simulink model "prjKGr_2021"  (R2023a)
settings: Solver=FixedStepAuto  StartTime=0.0  StopTime=60*5  FixedStep=0.002  RelTol=1e-3  EnableMultiTasking=on
values from neighbouring files (symbols this model uses):
  a0 = pi * (d0 / 2)^2    (= 1.55528471307e-05)    [calculate_matrix.m]    (also in equilibrum_h.m; param_G3.m)
  A0 = pi * (Di / 2)^2    (= 0.00155179165474)    [calculate_matrix.m]    (also in equilibrum_h.m; param_G3.m)
  A1 = pi * (Di / 2)^2    (= 0.00155179165474)    [calculate_matrix.m]    (also in equilibrum_h.m; param_G3.m)
  a1 = pi * (d1 / 2)^2    (= 2.42471809941e-05)    [calculate_matrix.m]    (also in equilibrum_h.m; param_G3.m)
  a2 = pi * (d0 / 2)^2    (= 1.55528471307e-05)    [calculate_matrix.m]    (also in equilibrum_h.m; param_G3.m)
  A2 = pi * (Di / 2)^2    (= 0.00155179165474)    [calculate_matrix.m]    (also in equilibrum_h.m; param_G3.m)
  A3 = pi * (Di / 2)^2    (= 0.00155179165474)    [calculate_matrix.m]    (also in equilibrum_h.m; param_G3.m)
  a3 = pi * (d1 / 2)^2    (= 2.42471809941e-05)    [calculate_matrix.m]    (also in equilibrum_h.m; param_G3.m)
  g = 9.8    [calculate_matrix.m]    (also in equilibrum_h.m; param_G3.m = 9.81)
  gamma = 0.61    [calculate_matrix.m]    (also in equilibrum_h.m; param_G3.m)
  h0eq = 0.1220    (= 0.122)    [param_G3.m]
  h1eq = 0.1286    [param_G3.m]
  h2eq = 0.1077    [param_G3.m]
  h3eq = 0.1252    [param_G3.m]
  K = -Quuinv*Qux    [param_G3.m]
  k0 = 3.9e-6    (= 3.9e-06)    [calculate_matrix.m]    (also in equilibrum_h.m; param_G3.m)
  k1 = 4.15e-6    (= 4.15e-06)    [calculate_matrix.m]    (also in equilibrum_h.m; param_G3.m)
  v0eq = 9.5    [param_G3.m]
  v1eq = 9.5    [param_G3.m]
undefined symbols (not defined in the file or in its folder): HIL
libraries: quarc_library x3
settings Model: Creator=Simulatore DELAB  LastModifiedBy=CRS
settings SolverCC: PositivePriorityOrder=on  AutoInsertRateTranBlk=on
settings DebuggingCC: UnconnectedInputMsg=warning  UnconnectedOutputMsg=warning  UnconnectedLineMsg=warning
settings ModelReferenceCC: EnableRefExpFcnMdlSchedulingChecks=on
settings RTWCC: Description=QUARC Win64 Target Using Toolchain  SystemTargetFile=quarc_win64.tlc  Toolchain=QUARC win64 | nmake (64-bit Windows)  BuildConfiguration=Faster Runs  DLArmComputeVersion=19.05
settings STFCustomTargetCC: SystemTargetFile=quarc_win64.tlc
settings GRTTargetCC: ParMdlRefBuildCompliant=off  CompOptLevelCompliant=off  CombineOutputUpdateFcns=off  MatFileLogging=off  CPPClassGenCompliant=off  GRTInterface=on  ExtMode=on  ExtModeMexFile=quarc_comm

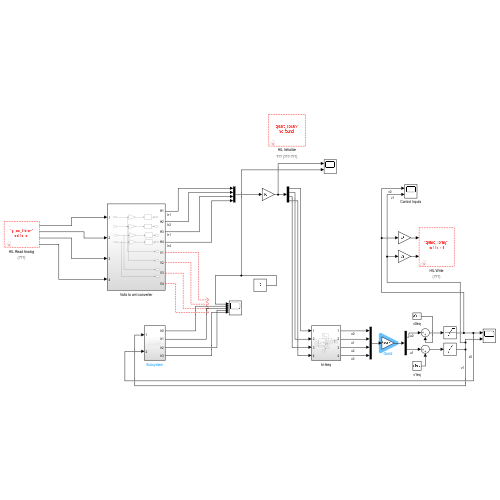
[thumbnail: Simulink's stored preview of the top-level diagram]
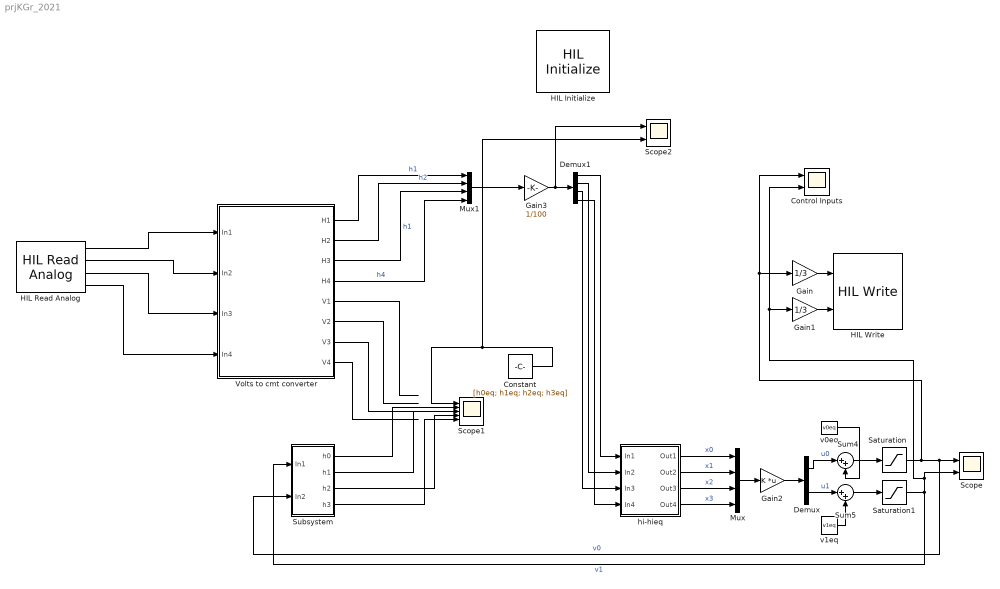
== system prjKGr_2021 ==
  Constant : Constant  Value=[h0eq; h1eq; h2eq; h3eq]
  Control Inputs : Scope  NumInputPorts=2
  Demux : Demux  Outputs=2
  Demux1 : Demux
  Gain : Gain  Gain=1/3
  Gain1 : Gain  Gain=1/3
  Gain2 : Gain  Gain=K  Multiplication=Matrix(K*u) (u vector)
  Gain3 : Gain  Gain=1/100
  HIL Initialize : quarc_library/Data Acquisition/Generic/Configuration/HIL Initialize  object_name=HIL-1  board_type=q8_usb  board_number=0  board_options=update_rate=normal;decimation=1  exclusive=off  active=on  hardware_clocks=[0:2]  clock_modes=[]  initial_clock_frequencies=[]  set_clock_params_at_start=off  set_clock_params_at_switch_in=off  set_clock_frequencies_at_start=off  set_clock_frequencies_at_switch_in=off  analog_input_channels=[0:7]  analog_input_configurations=[]  analog_input_maximums=10  analog_input_minimums=-10  set_analog_input_params_at_start=on  set_analog_input_params_at_switch_in=off  analog_output_channels=[0:7]  analog_output_maximums=10  analog_output_minimums=-10  initial_analog_outputs=[0]  final_analog_outputs=[0]  watchdog_analog_outputs=0  set_analog_output_params_at_start=on  set_analog_output_params_at_switch_in=off  set_analog_outputs_at_start=on  set_analog_outputs_at_switch_in=off  set_analog_outputs_at_terminate=on  set_analog_outputs_at_switch_out=off  set_analog_outputs_on_watchdog=off  digital_input_channels=[]  digital_output_channels=[]  digital_output_configuration=[]  initial_digital_outputs=[1]  final_digital_outputs=[1]  watchdog_digital_outputs=[1]  set_digital_output_params_at_start=off  set_digital_output_params_at_switch_in=off  set_digital_outputs_at_start=on  set_digital_outputs_at_switch_in=off  set_digital_outputs_at_terminate=on  set_digital_outputs_at_switch_out=off  set_digital_outputs_on_watchdog=off  encoder_channels=[0:7]  quadrature=[4]  encoder_filter_frequency=[]  initial_encoder_counts=[0]  set_encoder_params_at_start=on  set_encoder_params_at_switch_in=off  set_encoder_counts_at_start=on  set_encoder_counts_at_switch_in=off  pwm_channels=[0:7]  pwm_modes=0  pwm_frequency=99.532799999999995e6/4095  pwm_configuration=[0]  pwm_alignment=[0]  pwm_polarity=[1]  pwm_leading_deadband=[0]  pwm_trailing_deadband=[0]  initial_pwm_outputs=[0]  final_pwm_outputs=[0]  watchdog_pwm_outputs=[0]  set_pwm_params_at_start=on  set_pwm_params_at_switch_in=off  set_pwm_outputs_at_start=on  set_pwm_outputs_at_switch_in=off  set_pwm_outputs_at_terminate=on  set_pwm_outputs_at_switch_out=off  set_pwm_outputs_on_watchdog=off  other_output_channels=[]  initial_other_outputs=[]  final_other_outputs=[]  watchdog_other_outputs=[]  set_other_outputs_at_start=off  set_other_outputs_at_switch_in=off  set_other_outputs_at_terminate=off  set_other_outputs_at_switch_out=off  set_other_outputs_on_watchdog=off
  HIL Read Analog : quarc_library/Data Acquisition/Generic/Immediate I//O/HIL Read Analog  object_name=HIL-1  channels=0:3  sample_time=qc_get_step_size  active=on  vector_output=off
  HIL Write : quarc_library/Data Acquisition/Generic/Immediate I//O/HIL Write  object_name=HIL-1  analog_channels=0:1  pwm_channels=[]  digital_channels=[]  other_channels=[]  sample_time=-1  active=off  vector_input=off
  Mux : Mux
  Mux1 : Mux
  Saturation : Saturate  UpperLimit=15  LowerLimit=0
  Saturation1 : Saturate  UpperLimit=15  LowerLimit=0
  Scope : Scope  NumInputPorts=2
  Scope1 : Scope  NumInputPorts=5
  Scope2 : Scope  NumInputPorts=2
  Subsystem : Subsystem
  Sum4 : Sum  Inputs=|++
  Sum5 : Sum  Inputs=|++
  Volts to cmt converter : Subsystem
  hi-hieq : Subsystem
  v0eq : Constant  Value=v0eq
  v1eq : Constant  Value=v1eq
  wires:
  HIL Read Analog/1 -> Volts to cmt converter/1(In1)
  HIL Read Analog/2 -> Volts to cmt converter/2(In2)
  HIL Read Analog/3 -> Volts to cmt converter/3(In3)
  HIL Read Analog/4 -> Volts to cmt converter/4(In4)
  Volts to cmt converter/5(V1) -> ?
  Volts to cmt converter/6(V2) -> ?
  Volts to cmt converter/7(V3) -> ?
  Volts to cmt converter/8(V4) -> ?
  Gain/1 -> HIL Write/1
  Gain1/1 -> HIL Write/2
  Volts to cmt converter/1(H1) -> Mux1/1  "h1"
  Volts to cmt converter/2(H2) -> Mux1/2  "h2"
  Volts to cmt converter/3(H3) -> Mux1/3  "h1"
  Volts to cmt converter/4(H4) -> Mux1/4  "h4"
  Constant/1 -> Scope2/2, Scope1/1
  Subsystem/3(h2) -> Scope1/4
  Subsystem/1(h0) -> Scope1/2
  hi-hieq/1(Out1) -> Mux/1  "x0"
  Saturation/1 -> Control Inputs/1, Gain/1, Subsystem/2(In2), Scope/1  "v0"
  hi-hieq/2(Out2) -> Mux/2  "x1"
  hi-hieq/4(Out4) -> Mux/4  "x3"
  Subsystem/4(h3) -> Scope1/5
  hi-hieq/3(Out3) -> Mux/3  "x2"
  Subsystem/2(h1) -> Scope1/3
  Sum5/1 -> Saturation1/1
  Gain2/1 -> Demux/1
  v0eq/1 -> Sum4/2
  Saturation1/1 -> Control Inputs/2, Gain1/1, Scope/2, Subsystem/1(In1)  "v1"
  Demux/2 -> Sum5/1  "u1"
  v1eq/1 -> Sum5/2
  Sum4/1 -> Saturation/1
  Demux/1 -> Sum4/1  "u0"
  Mux/1 -> Gain2/1
  Mux1/1 -> Gain3/1
  Gain3/1 -> Scope2/1, Demux1/1
  Demux1/1 -> hi-hieq/1(In1)
  Demux1/2 -> hi-hieq/2(In2)
  Demux1/3 -> hi-hieq/3(In3)
  Demux1/4 -> hi-hieq/4(In4)

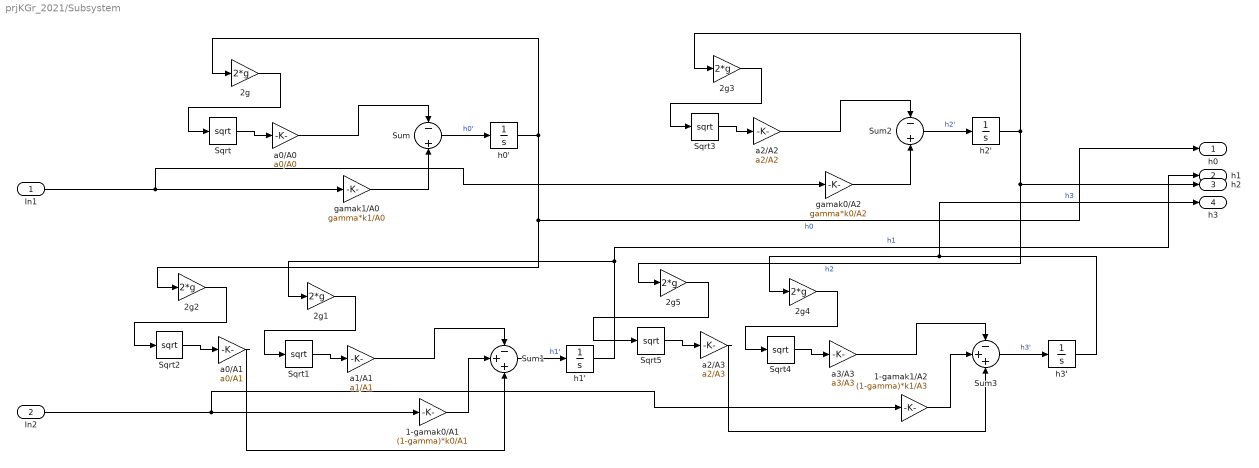
== system prjKGr_2021/Subsystem ==
  In1 : Inport
  In2 : Inport  Port=2
  1-gamak0/A1 : Gain  Gain=(1-gamma)*k0/A1
  1-gamak1/A2 : Gain  Gain=(1-gamma)*k1/A3
  2g{,1..5} (6 alike) : Gain  Gain=2*g
  Sqrt{,1..5} (6 alike) : Sqrt
  Sum : Sum  Inputs=-+
  Sum1 : Sum  Inputs=-++
  Sum2 : Sum  Inputs=-+
  Sum3 : Sum  Inputs=-++
  a0/A0 : Gain  Gain=a0/A0
  a0/A1 : Gain  Gain=a0/A1
  a1/A1 : Gain  Gain=a1/A1
  a2/A2 : Gain  Gain=a2/A2
  a2/A3 : Gain  Gain=a2/A3
  a3/A3 : Gain  Gain=a3/A3
  gamak0/A2 : Gain  Gain=gamma*k0/A2
  gamak1/A0 : Gain  Gain=gamma*k1/A0
  h0' : Integrator
  h1' : Integrator
  h2' : Integrator
  h3' : Integrator
  h0 : Outport
  h1 : Outport  Port=2
  h2 : Outport  Port=3
  h3 : Outport  Port=4
  wires:
  h3'/1 -> 2g4/1, h3/1  "h3"
  Sum1/1 -> h1'/1  "h1'"
  2g/1 -> Sqrt/1
  Sum/1 -> h0'/1  "h0'"
  a3/A3/1 -> Sum3/1
  h0'/1 -> 2g/1, h0/1, 2g2/1  "h0"
  1-gamak0/A1/1 -> Sum1/2
  gamak1/A0/1 -> Sum/2
  2g2/1 -> Sqrt2/1
  Sqrt1/1 -> a1/A1/1
  2g5/1 -> Sqrt5/1
  a1/A1/1 -> Sum1/1
  a0/A0/1 -> Sum/1
  h2'/1 -> h2/1, 2g5/1, 2g3/1  "h2"
  Sqrt5/1 -> a2/A3/1
  Sum3/1 -> h3'/1  "h3'"
  In2/1 -> 1-gamak1/A2/1, 1-gamak0/A1/1
  1-gamak1/A2/1 -> Sum3/2
  a2/A3/1 -> Sum3/3
  h1'/1 -> h1/1, 2g1/1  "h1"
  2g4/1 -> Sqrt4/1
  Sqrt2/1 -> a0/A1/1
  a2/A2/1 -> Sum2/1
  Sqrt4/1 -> a3/A3/1
  Sqrt/1 -> a0/A0/1
  2g3/1 -> Sqrt3/1
  2g1/1 -> Sqrt1/1
  gamak0/A2/1 -> Sum2/2
  Sum2/1 -> h2'/1  "h2'"
  a0/A1/1 -> Sum1/3
  Sqrt3/1 -> a2/A2/1
  In1/1 -> gamak0/A2/1, gamak1/A0/1

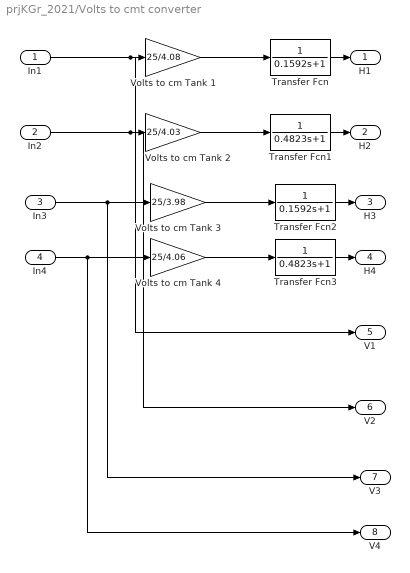
== system prjKGr_2021/Volts to cmt converter ==
  In1 : Inport
  In2 : Inport  Port=2
  In3 : Inport  Port=3
  In4 : Inport  Port=4
  Transfer Fcn : TransferFcn  Denominator=[0.1592 1]
  Transfer Fcn1 : TransferFcn  Denominator=[0.4823 1]
  Transfer Fcn2 : TransferFcn  Denominator=[0.1592 1]
  Transfer Fcn3 : TransferFcn  Denominator=[0.4823 1]
  Volts to cm Tank 1 : Gain  Gain=25/4.08
  Volts to cm Tank 2 : Gain  Gain=25/4.03
  Volts to cm Tank 3 : Gain  Gain=25/3.98
  Volts to cm Tank 4 : Gain  Gain=25/4.06
  H1 : Outport
  H2 : Outport  Port=2
  H3 : Outport  Port=3
  H4 : Outport  Port=4
  V1 : Outport  Port=5
  V2 : Outport  Port=6
  V3 : Outport  Port=7
  V4 : Outport  Port=8
  wires:
  Volts to cm Tank 1/1 -> Transfer Fcn/1
  Volts to cm Tank 3/1 -> Transfer Fcn2/1
  In4/1 -> V4/1, Volts to cm Tank 4/1
  Transfer Fcn3/1 -> H4/1
  Volts to cm Tank 4/1 -> Transfer Fcn3/1
  Volts to cm Tank 2/1 -> Transfer Fcn1/1
  In2/1 -> V2/1, Volts to cm Tank 2/1
  In3/1 -> V3/1, Volts to cm Tank 3/1
  Transfer Fcn2/1 -> H3/1
  Transfer Fcn1/1 -> H2/1
  Transfer Fcn/1 -> H1/1
  In1/1 -> V1/1, Volts to cm Tank 1/1

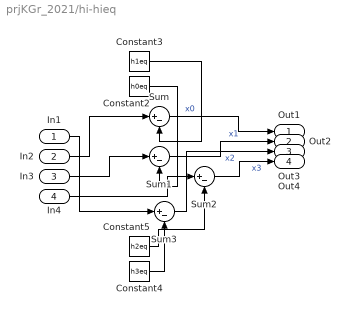
== system prjKGr_2021/hi-hieq ==
  In1 : Inport
  In2 : Inport  Port=2
  In3 : Inport  Port=3
  In4 : Inport  Port=4
  Constant2 : Constant  Value=h0eq
  Constant3 : Constant  Value=h1eq
  Constant4 : Constant  Value=h3eq
  Constant5 : Constant  Value=h2eq
  Sum{,1..3} (4 alike) : Sum  Inputs=|+-
  Out1 : Outport
  Out2 : Outport  Port=2
  Out3 : Outport  Port=3
  Out4 : Outport  Port=4
  wires:
  In2/1 -> Sum/1
  Constant5/1 -> Sum2/2
  Constant3/1 -> Sum/2
  Sum1/1 -> Out2/1  "x1"
  Constant4/1 -> Sum3/2
  In1/1 -> Sum3/1
  Constant2/1 -> Sum1/2
  In4/1 -> Sum2/1
  In3/1 -> Sum1/1
  Sum/1 -> Out1/1  "x0"
  Sum2/1 -> Out4/1  "x3"
  Sum3/1 -> Out3/1  "x2"
